simulink model "nn_gensim"  (R2020a)
settings: Solver=VariableStepAuto  StartTime=0.0  StopTime=10.0  RelTol=1e-3
libraries: neural x67
(part 5 of 5)

== system nn_gensim/Feed-Forward Neural Network/Layer 3/Delays 1 ==
  "p{3}" : Inport  PortDimensions=30
      mask Display: e = 0.06;c1 = [120 230 180]/255;c2 = ([120 230 180]+0)/(256+128);c3 = ([120 230 180]+128)/(256+128);patch([0 1 1 0],[0 0 1 1],c1);patch([0 1 1 1-e 1-e 0+e],[0 0 1 1-e 0+e 0+e],c2);patch([0 0 1 1-e 0+e 0+e],[0 1 1 1-e 1-e 0+e],c3);plot([0 1 1 0 0],[0 0 1 1 0]);
  mux : Mux  Inputs=1
      mask Display: e = 0.06;c1 = [120 150 230]/255;c2 = ([120 150 230]+0)/383;c3 = ([120 150 230]+128)/383;patch([0 1 1 0],[0 0 1 1],c1);patch([0 1 1 1-e 1-e 0+e],[0 0 1 1-e 0+e 0+e],c2);patch([0 0 1 1-e 0+e 0+e],[0 1 1 1-e 1-e 0+e],c3);plot([0 1 1 0 0],[0 0 1 1 0]);disp('Mux')
  "pd{3,2}" : Outport
      mask Display: e = 0.06;c1 = [120 230 180]/255;c2 = ([120 230 180]+0)/(256+128);c3 = ([120 230 180]+128)/(256+128);patch([0 1 1 0],[0 0 1 1],c1);patch([0 1 1 1-e 1-e 0+e],[0 0 1 1-e 0+e 0+e],c2);patch([0 0 1 1-e 0+e 0+e],[0 1 1 1-e 1-e 0+e],c3);plot([0 1 1 0 0],[0 0 1 1 0]);
  wires:
  "p{3}"/1 -> mux/1
  mux/1 -> "pd{3,2}"/1

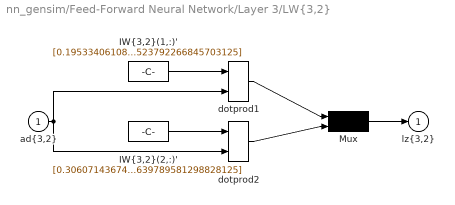
== system nn_gensim/Feed-Forward Neural Network/Layer 3/LW{3,2} ==
  "ad{3,2}" : Inport  PortDimensions=30
      mask Display: e = 0.06;c1 = [120 230 180]/255;c2 = ([120 230 180]+0)/(256+128);c3 = ([120 230 180]+128)/(256+128);patch([0 1 1 0],[0 0 1 1],c1);patch([0 1 1 1-e 1-e 0+e],[0 0 1 1-e 0+e 0+e],c2);patch([0 0 1 1-e 0+e 0+e],[0 1 1 1-e 1-e 0+e],c3);plot([0 1 1 0 0],[0 0 1 1 0]);
  "IW{3,2}(1,:)'" : Constant  Value=[0.1953340610836440394137980547384358942508697509765625;-0.1834169876427222956039031487307511270046234130859375;-0.6401306263873898227956260598148219287395477294921875;-0.9864844567093913330069199218996800482273101806640625;0.4089393627757214044748934611561708152294158935546875;0.4329778492439648740486290989792905747890472412109375;0.33053921532659114035368475015275180339813232421875;-0.04059640493436145192163166939280927181243896484375;-0.8522795693394320526437013540999032557010650634765625;-0.2773537160204628815307614786433987319469451904296875;0.6185247037069754316718217523884959518909454345703125;-0.2068951450717888551622536397189833223819732666015625;0.9683308366795218002920364597230218350887298583984375;0.67823319891556455019099303171969950199127197265625;-0.1067167673769089386581754297367297112941741943359375;-0.1460482946721153307834129009279422461986541748046875;-0.029272377952965111802541287033818662166595458984375;-0.5157241716168019518562459779786877334117889404296875;-0.6963218352197599880781808678875677287578582763671875;0.759909516928374717537053584237582981586456298828125;-0.0489163986664127303782834133016876876354217529296875;0.745250714641694234074975611292757093906402587890625;0.6693495662634088017028943795594386756420135498046875;0.7819846524506584017899513128213584423065185546875;0.1659236182465393394380726022063754498958587646484375;0.386103999850855306164021385484375059604644775390625;0.3504853394226514762266333491425029933452606201171875;0.3213430273208526255501737978192977607250213623046875;0.237559903461370236499305974575690925121307373046875;-0.97389739323054147490665855002589523792266845703125]
      mask Display: e = 0.06;c1 = [120 150 230]/255;c2 = ([120 150 230]+0)/383;c3 = ([120 150 230]+128)/383;patch([0 1 1 0],[0 0 1 1],c1);patch([0 1 1 1-e 1-e 0+e],[0 0 1 1-e 0+e 0+e],c2);patch([0 0 1 1-e 0+e 0+e],[0 1 1 1-e 1-e 0+e],c3);plot([0 1 1 0 0],[0 0 1 1 0]);disp('weights');
  "IW{3,2}(2,:)'" : Constant  Value=[0.3060714367408350344845757717848755419254302978515625;0.2394214839820474338694111793301999568939208984375;0.454224099086458554808132248581387102603912353515625;-0.131034430518865985249021832714788615703582763671875;-0.005533190882461180848395088105462491512298583984375;0.9336642621913531225885662934160791337490081787109375;0.0947134392396138391490012509166263043880462646484375;-0.5704863347418120955722997678094543516635894775390625;0.1324077427214300772817523466073907911777496337890625;-0.5889014967293280111704234514036215841770172119140625;0.4205711814323624953004809867707081139087677001953125;-0.5828566082714663476593841551220975816249847412109375;-0.5682322141682758509517725542536936700344085693359375;0.079555311242202275678891965071670711040496826171875;-0.936272092617877138565063432906754314899444580078125;-0.362923915829000964805572948534972965717315673828125;0.12128586329696844359204987995326519012451171875;-0.0769761571237681518908857469796203076839447021484375;-0.1922939520976958416298430165625177323818206787109375;0.6966473131460213519261515102698467671871185302734375;0.240145239913344799020933351130224764347076416015625;-0.7315571597784440438516639915178529918193817138671875;-0.748885565355299487322326967841945588588714599609375;-0.047993010657776391525430881301872432231903076171875;-0.851897480795091865957147092558443546295166015625;-0.5779267890074830660296356654725968837738037109375;-0.1150313857236244796666824186104349792003631591796875;0.2456619454877724262331639693002216517925262451171875;-0.4947448025908347535306575082358904182910919189453125;-0.4195217981868737400219515620847232639789581298828125]
      mask Display: e = 0.06;c1 = [120 150 230]/255;c2 = ([120 150 230]+0)/383;c3 = ([120 150 230]+128)/383;patch([0 1 1 0],[0 0 1 1],c1);patch([0 1 1 1-e 1-e 0+e],[0 0 1 1-e 0+e 0+e],c2);patch([0 0 1 1-e 0+e 0+e],[0 1 1 1-e 1-e 0+e],c3);plot([0 1 1 0 0],[0 0 1 1 0]);disp('weights');
  Mux : Mux  Inputs=2
      mask Display: e = 0.06;c1 = [120 150 230]/255;c2 = ([120 150 230]+0)/383;c3 = ([120 150 230]+128)/383;patch([0 1 1 0],[0 0 1 1],c1);patch([0 1 1 1-e 1-e 0+e],[0 0 1 1-e 0+e 0+e],c2);patch([0 0 1 1-e 0+e 0+e],[0 1 1 1-e 1-e 0+e],c3);plot([0 1 1 0 0],[0 0 1 1 0]);disp('Mux');
  dotprod1 : neural/Weight Functions/dotprod
  dotprod2 : neural/Weight Functions/dotprod
  "lz{3,2}" : Outport
      mask Display: e = 0.06;c1 = [120 230 180]/255;c2 = ([120 230 180]+0)/(256+128);c3 = ([120 230 180]+128)/(256+128);patch([0 1 1 0],[0 0 1 1],c1);patch([0 1 1 1-e 1-e 0+e],[0 0 1 1-e 0+e 0+e],c2);patch([0 0 1 1-e 0+e 0+e],[0 1 1 1-e 1-e 0+e],c3);plot([0 1 1 0 0],[0 0 1 1 0]);
  wires:
  "IW{3,2}(1,:)'"/1 -> dotprod1/1
  "ad{3,2}"/1 -> dotprod1/2, dotprod2/2
  dotprod1/1 -> Mux/1
  "IW{3,2}(2,:)'"/1 -> dotprod2/1
  dotprod2/1 -> Mux/2
  Mux/1 -> "lz{3,2}"/1
